simulink model "FSFB_FF_HIL"  (R2022a)
settings: Solver=FixedStepAuto  StartTime=0.0  StopTime=500  FixedStep=0.0001  RelTol=1e-9
settings Model: SimulationMode=external  Creator=zachn  LastModifiedBy=domin
settings SolverCC: AlgebraicLoopSolver=TrustRegion
settings DataIOCC: SaveFormat=StructureWithTime  InspectSignalLogs=on
settings DebuggingCC: UnconnectedInputMsg=warning  UnconnectedOutputMsg=warning  UnconnectedLineMsg=warning  SFMachineParentedDataDiag=warning
settings HardwareCC: ProdBitPerLong=64  ProdHWDeviceType=Intel->x86-64 (Linux 64)
settings RTWCC: Description=Simulink Desktop Real-Time  SystemTargetFile=sldrt.tlc  TemplateMakefile=sldrt.tmf  RTWCompilerOptimization=on  DLArmComputeVersion=19.05
settings CodeAppCC: MaxIdLength=95
settings SimulinkDesktopRealTimeCC: TargetLibSuffix=_sldrt.a  TargetPreCompLibLocation=C:\Program Files\MATLAB\R2022a\toolbox\sldrt\lib\win64

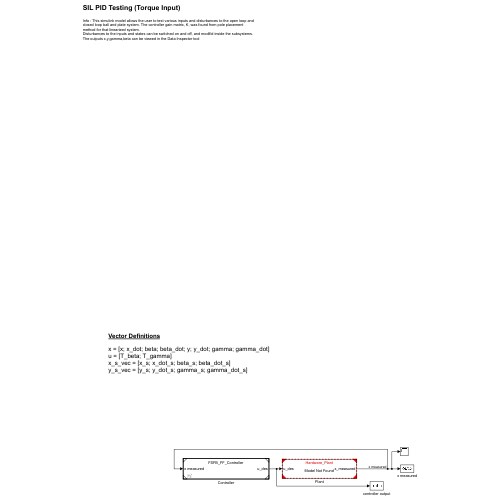
[thumbnail: Simulink's stored preview of the top-level diagram]
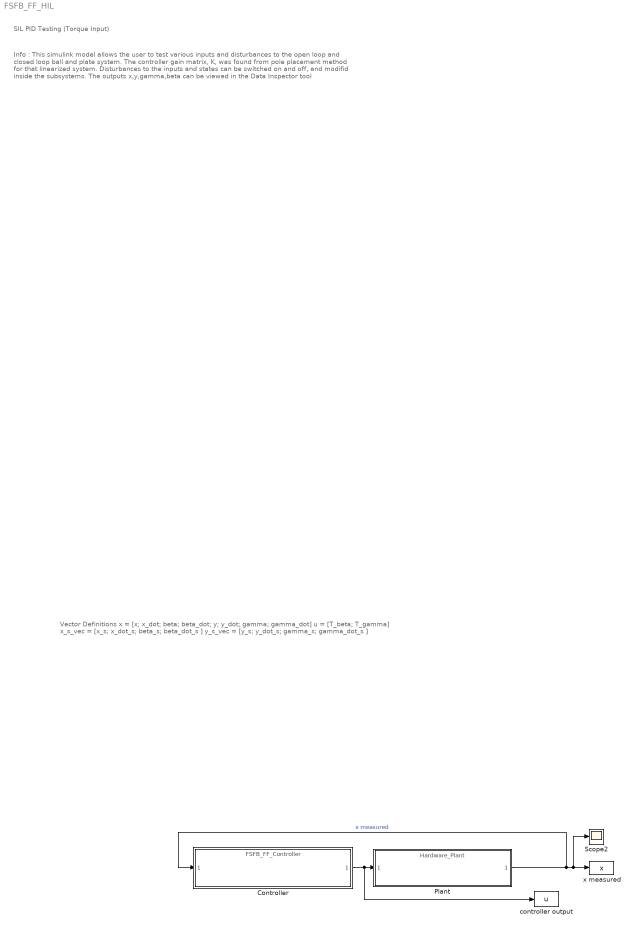
== system FSFB_FF_HIL ==
  note: Info : This simulink model allows the user to test various inputs and disturbances to the open loop and closed loop ball and plate system. The controller gain matrix, K, was found from pole placement
      | method for that linearized system.
      | Disturbances to the inputs and states can be switched on and off, and modifid inside the subsystems.
      | The outputs x,y,gamma,beta can be viewed in the Data Inspector tool
  note: SIL PID Testing (Torque Input)
  note: Vector Definitions
      |
      | x = [x; x_dot; beta; beta_dot; y; y_dot; gamma; gamma_dot]
      | u = [T_beta; T_gamma]
      | x_s_vec = [x_s; x_dot_s; beta_s; beta_dot_s ]
      | y_s_vec = [y_s; y_dot_s; gamma_s; gamma_dot_s ]
  Controller : ModelReference  ModelNameDialog=FSFB_FF_Controller  SimulationMode=Normal  ModelReferenceVersion=1.22
  Plant : ModelReference  ModelNameDialog=Hardware_Plant  SimulationMode=Normal  ModelReferenceVersion=5.35
  Scope2 : Scope
  controller output : ToWorkspace  VariableName=u  SampleTime=-1
  x measured : ToWorkspace  VariableName=x  SampleTime=-1
  wires:
  Controller/1 -> controller output/1, Plant/1
  Plant/1 -> Controller/1, Scope2/1, x measured/1  "x measured"
